simulink model "scdspeed"  (Simulink 6.0)
settings: Solver=ode23  StartTime=0.0  StopTime=10  FixedStep=0.1  MaxStep=0.01  RelTol=1e-3
model workspace (MAT data in the model file):
  p = [-7.82997288351e-05; 0.181210895977; -0.072497134344; 0.000486358314052; 0.0361674637937]
settings Model: Creator=jglass  LastModifiedBy=jglass  BufferReuse=off
settings DataIOCC: SignalLoggingName=logsOut
settings OptimizationCC: InlineParams=on  BufferReuse=off
settings DebuggingCC: CheckExecutionContextPreStartOutputMsg=on  CheckExecutionContextRuntimeOutputMsg=on  SolverPrmCheckMsg=none

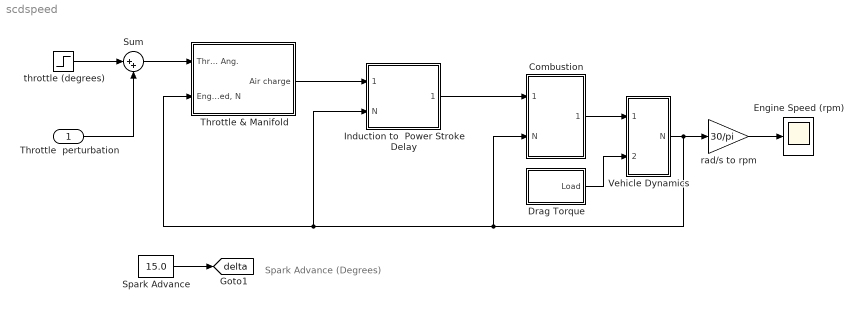
== system scdspeed ==
  note: Spark Advance
      | (Degrees)
  Throttle  perturbation : Inport  LatchInput=off
  Combustion : Subsystem  PropExecContextAcrossSSBoundary=on
  Drag Torque : Subsystem  PropExecContextAcrossSSBoundary=on
  Engine Speed (rpm) : Scope
      settings: TickLabels=on  TimeRange=10  YMin=1500  YMax=3500  SaveName=N  DataFormat=Structure
  Induction to  Power Stroke Delay : Subsystem  PropExecContextAcrossSSBoundary=on
  Spark Advance : Constant  Value=15.0
  Sum : Sum  Inputs=|++
  Throttle & Manifold : Subsystem  PropExecContextAcrossSSBoundary=on
  Vehicle Dynamics : Subsystem  PropExecContextAcrossSSBoundary=on
  rad/s to rpm : Gain  Gain=30/pi  SaturateOnIntegerOverflow=on
  throttle (degrees) : Step  Time=2  Before=8.973  After=11  SampleTime=0
  tag scope: delta=global
  wires:
  Throttle & Manifold/1(Air charge) -> Induction to  Power Stroke Delay/1(Air charge)
  Vehicle Dynamics/1(N) -> Combustion/2(N), Throttle & Manifold/2("Engine Speed, N"), Induction to  Power Stroke Delay/2(N), rad/s to rpm/1
  rad/s to rpm/1 -> Engine Speed (rpm)/1
  Combustion/1(Torque) -> Vehicle Dynamics/1(Teng)
  Drag Torque/1(Load) -> Vehicle Dynamics/2(Tload)
  Spark Advance/1 -> [delta]
  Induction to  Power Stroke Delay/1(Air Charge) -> Combustion/1(Air Charge)
  throttle (degrees)/1 -> Sum/1
  Sum/1 -> Throttle & Manifold/1(Throttle Ang.)
  Throttle  perturbation/1 -> Sum/2

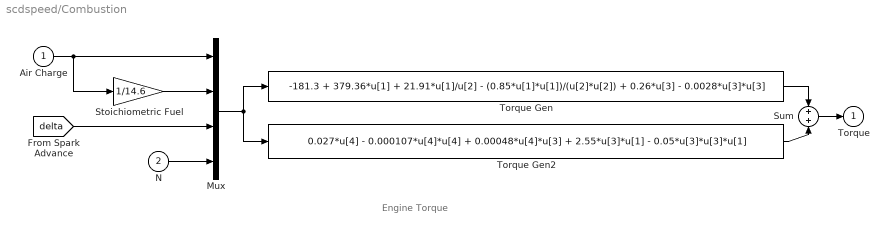
== system scdspeed/Combustion ==
  note: Engine Torque
  Air Charge : Inport  LatchInput=off
  N : Inport  Port=2  LatchInput=off
  Mux : Mux
  Stoichiometric Fuel : Gain  Gain=1/14.6  SaturateOnIntegerOverflow=on
  Sum : Sum  SaturateOnIntegerOverflow=on  InputSameDT=on
  Torque Gen : Fcn  Expr=-181.3 + 379.36*u[1] + 21.91*u[1]/u[2] - (0.85*u[1]*u[1])/(u[2]*u[2]) + 0.26*u[3] - 0.0028*u[3]*u[3]
  Torque Gen2 : Fcn  Expr=0.027*u[4] - 0.000107*u[4]*u[4] + 0.00048*u[4]*u[3] + 2.55*u[3]*u[1] - 0.05*u[3]*u[3]*u[1]
  Torque : Outport  InitialOutput=0
  wires:
  Stoichiometric Fuel/1 -> Mux/2
  [delta] -> Mux/3
  N/1 -> Mux/4
  Air Charge/1 -> Stoichiometric Fuel/1, Mux/1
  Mux/1 -> Torque Gen/1, Torque Gen2/1
  Torque Gen2/1 -> Sum/2
  Torque Gen/1 -> Sum/1
  Sum/1 -> Torque/1

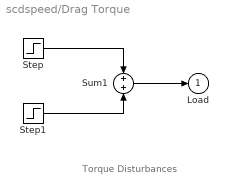
== system scdspeed/Drag Torque ==
  note: Torque Disturbances
  Step : Step  Time=2  Before=25  After=25  SampleTime=0
  Step1 : Step  Time=8  After=0  SampleTime=0
  Sum1 : Sum  SaturateOnIntegerOverflow=on  InputSameDT=on
  Load : Outport  InitialOutput=0
  wires:
  Step1/1 -> Sum1/2
  Step/1 -> Sum1/1
  Sum1/1 -> Load/1

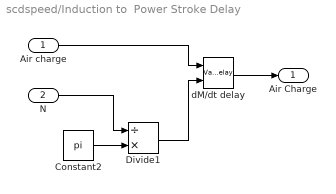
== system scdspeed/Induction to  Power Stroke Delay ==
  Air charge : Inport  LatchInput=off
  N : Inport  Port=2  LatchInput=off
  Constant2 : Constant  Value=pi
  Divide1 : Product  Inputs=/*  OutScaling=2^-10
  dM/dt delay : VariableTransportDelay  MaximumDelay=10  InitialInput=0.152  PadeOrder=2  TransDelayFeedthrough=on
  Air Charge : Outport
  wires:
  dM/dt delay/1 -> Air Charge/1
  Constant2/1 -> Divide1/2
  N/1 -> Divide1/1
  Divide1/1 -> dM/dt delay/2
  Air charge/1 -> dM/dt delay/1

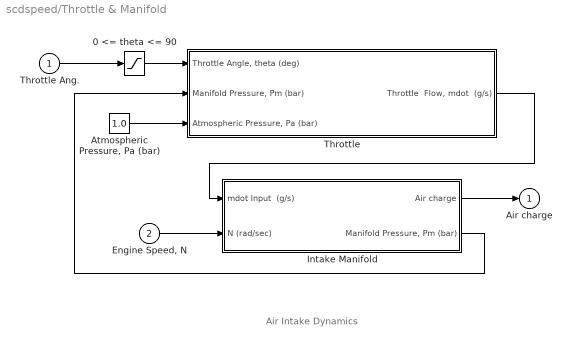
== system scdspeed/Throttle & Manifold ==
  note: Air Intake Dynamics
  Throttle Ang. : Inport  LatchInput=off
  "Engine Speed, N" : Inport  Port=2  LatchInput=off
  0 <= theta <= 90 : Saturate  UpperLimit=90  LowerLimit=0
  "Atmospheric Pressure, Pa (bar)" : Constant  Value=1.0
  Intake Manifold : Subsystem  PropExecContextAcrossSSBoundary=on
  Throttle : Subsystem  PropExecContextAcrossSSBoundary=on
  Air charge : Outport  InitialOutput=0
  wires:
  "Atmospheric Pressure, Pa (bar)"/1 -> Throttle/3("Atmospheric Pressure, Pa (bar) ")
  Intake Manifold/1(Air charge) -> Air charge/1
  Intake Manifold/2("Manifold Pressure, Pm (bar)") -> Throttle/2("Manifold Pressure, Pm (bar)")
  "Engine Speed, N"/1 -> Intake Manifold/2(N (rad/sec))
  Throttle/1("Throttle  Flow, mdot  (g/s)") -> Intake Manifold/1(mdot Input  (g/s))
  Throttle Ang./1 -> 0 <= theta <= 90/1
  0 <= theta <= 90/1 -> Throttle/1("Throttle Angle, theta (deg)")

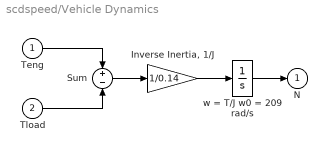
== system scdspeed/Vehicle Dynamics ==
  Teng : Inport  LatchInput=off
  Tload : Inport  Port=2  LatchInput=off
  "Inverse Inertia, 1/J" : Gain  Gain=1/0.14  SaturateOnIntegerOverflow=on
  Sum : Sum  Inputs=+-  SaturateOnIntegerOverflow=on  InputSameDT=on
  w = T/J w0 = 209 rad/s : Integrator  InitialCondition=209.48
  N : Outport  InitialOutput=0
  wires:
  "Inverse Inertia, 1/J"/1 -> w = T/J w0 = 209 rad/s/1
  w = T/J w0 = 209 rad/s/1 -> N/1
  Sum/1 -> "Inverse Inertia, 1/J"/1
  Teng/1 -> Sum/1
  Tload/1 -> Sum/2

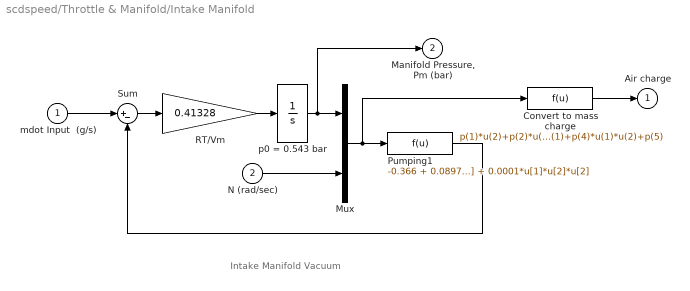
== system scdspeed/Throttle & Manifold/Intake Manifold ==
  note: Intake Manifold Vacuum
  mdot Input  (g/s) : Inport  LatchInput=off
  N (rad/sec) : Inport  Port=2  LatchInput=off
  Convert to mass charge : Fcn  Expr=p(1)*u(2)+p(2)*u(1)+p(3)*u(1)*u(1)+p(4)*u(1)*u(2)+p(5)
  Mux : Mux  Inputs=2
  Pumping1 : Fcn  Expr=-0.366 + 0.08979*u[1]*u[2] - 0.0337*u[2]*u[1]*u[1] + 0.0001*u[1]*u[2]*u[2]
  RT/Vm : Gain  Gain=0.41328  SaturateOnIntegerOverflow=on
  Sum : Sum  Inputs=|+-  SaturateOnIntegerOverflow=on  InputSameDT=on
  p0 = 0.543 bar : Integrator  InitialCondition=.543
  Air charge : Outport  InitialOutput=0
  "Manifold Pressure, Pm (bar)" : Outport  Port=2  InitialOutput=0
  wires:
  Pumping1/1 -> Sum/2
  Sum/1 -> RT/Vm/1
  p0 = 0.543 bar/1 -> "Manifold Pressure, Pm (bar)"/1, Mux/1
  Mux/1 -> Pumping1/1, Convert to mass charge/1
  N (rad/sec)/1 -> Mux/2
  RT/Vm/1 -> p0 = 0.543 bar/1
  mdot Input  (g/s)/1 -> Sum/1
  Convert to mass charge/1 -> Air charge/1

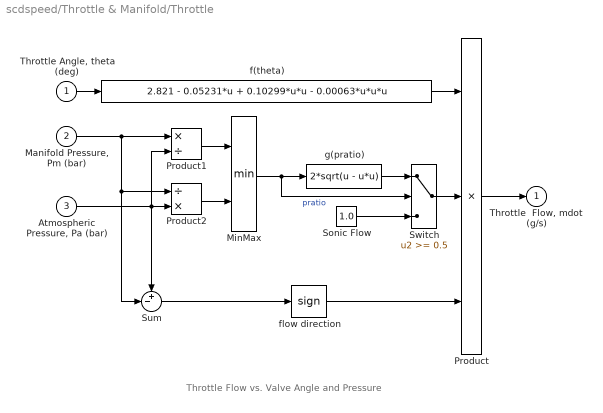
== system scdspeed/Throttle & Manifold/Throttle ==
  note: Throttle Flow vs. Valve Angle and Pressure
  "Throttle Angle, theta (deg)" : Inport  LatchInput=off
  "Manifold Pressure, Pm (bar)" : Inport  Port=2  LatchInput=off
  "Atmospheric Pressure, Pa (bar) " : Inport  Port=3  LatchInput=off
  MinMax : MinMax  Inputs=2  SaturateOnIntegerOverflow=on  InputSameDT=on
  Product : Product  Inputs=3  SaturateOnIntegerOverflow=on  RndMeth=Zero  InputSameDT=on
  Product1 : Product  Inputs=*/  SaturateOnIntegerOverflow=on  RndMeth=Zero  InputSameDT=on
  Product2 : Product  Inputs=/*  SaturateOnIntegerOverflow=on  RndMeth=Zero  InputSameDT=on
  "Sonic Flow " : Constant  Value=1.0
  Sum : Sum  Inputs=+-|  SaturateOnIntegerOverflow=on  InputSameDT=on
  Switch : Switch  Threshold=0.5  SaturateOnIntegerOverflow=on  InputSameDT=on
  f(theta) : Fcn  Expr=2.821 - 0.05231*u + 0.10299*u*u - 0.00063*u*u*u
  flow direction : Signum
  g(pratio) : Fcn  Expr=2*sqrt(u - u*u)
  "Throttle  Flow, mdot  (g/s)" : Outport  InitialOutput=0
  wires:
  f(theta)/1 -> Product/1
  Product/1 -> "Throttle  Flow, mdot  (g/s)"/1
  "Throttle Angle, theta (deg)"/1 -> f(theta)/1
  MinMax/1 -> g(pratio)/1, Switch/2  "pratio"
  Sum/1 -> flow direction/1
  flow direction/1 -> Product/3
  Switch/1 -> Product/2
  "Sonic Flow "/1 -> Switch/3
  g(pratio)/1 -> Switch/1
  "Atmospheric Pressure, Pa (bar) "/1 -> Product1/2, Product2/2, Sum/1
  Product1/1 -> MinMax/1
  Product2/1 -> MinMax/2
  "Manifold Pressure, Pm (bar)"/1 -> Product1/1, Product2/1, Sum/2
